simulink model "Gain"  (R2017b)
settings: Solver=FixedStepDiscrete  StartTime=0.0  StopTime=10.0  FixedStep=0.200000  RelTol=1e-3
settings Model: Creator=hbourbou  LastModifiedBy=hbourbou
settings DataIOCC: SaveFormat=StructureWithTime
settings OptimizationCC: LifeSpan=inf
settings DebuggingCC: SFExecutionAtInitializationDiag=none
settings HardwareCC: ProdBitPerSizeT=32  ProdBitPerPtrDiffT=32  ProdWordSize=32  ProdHWDeviceType=Specified
settings CodeAppCC: StateflowObjectComments=on

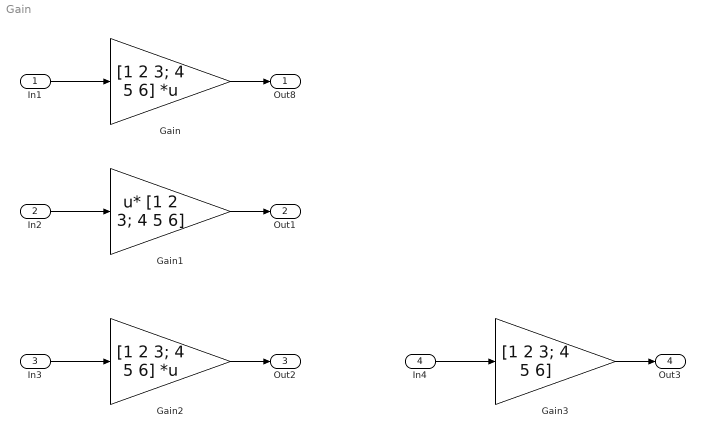
== system Gain ==
  In1 : Inport  PortDimensions=[3 2]
  In2 : Inport  Port=2  PortDimensions=[3 2]
  In3 : Inport  Port=3  PortDimensions=3
  In4 : Inport  Port=4  PortDimensions=[2 3]
  Gain : Gain  Gain=[1 2 3; 4 5 6]  Multiplication=Matrix(K*u)
  Gain1 : Gain  Gain=[1 2 3; 4 5 6]  Multiplication=Matrix(u*K)
  Gain2 : Gain  Gain=[1 2 3; 4 5 6]  Multiplication=Matrix(K*u) (u vector)
  Gain3 : Gain  Gain=[1 2 3; 4 5 6]
  Out8 : Outport
  Out1 : Outport  Port=2
  Out2 : Outport  Port=3
  Out3 : Outport  Port=4
  wires:
  In1/1 -> Gain/1
  Gain/1 -> Out8/1
  In2/1 -> Gain1/1
  Gain1/1 -> Out1/1
  In3/1 -> Gain2/1
  Gain2/1 -> Out2/1
  In4/1 -> Gain3/1
  Gain3/1 -> Out3/1
